simulink model "Forward_Kinematic"  (R2016a)
settings: Solver=VariableStepAuto  StartTime=0.0  StopTime=5  RelTol=1e-3
values from neighbouring files (symbols this model uses):
  l1 = 315    [FORWARD_KINEMATICS_DELTA_ROBOT.m]    (also in Inverse_Dynamic_Model.m = 0.1; Kinematic_Dimension.m = 0.315; inverse_kinematic.m = 0.1)
  phi = [phi1; phi2; phi3]    [Inverse_Dynamic_Model.m]    (also in Kinematic_Dimension.m; inverse_kinematic.m)
  r1 = 225    [FORWARD_KINEMATICS_DELTA_ROBOT.m]    (also in Inverse_Dynamic_Model.m = 0.35; Kinematic_Dimension.m = 0.225; inverse_kinematic.m = 0.35)
  r2 = 75    [FORWARD_KINEMATICS_DELTA_ROBOT.m]    (also in Inverse_Dynamic_Model.m = 0.35; Kinematic_Dimension.m = 0.075; inverse_kinematic.m = 0.35)
settings Model: Creator=computer  LastModifiedBy=computer
settings DataIOCC: SaveFormat=Array

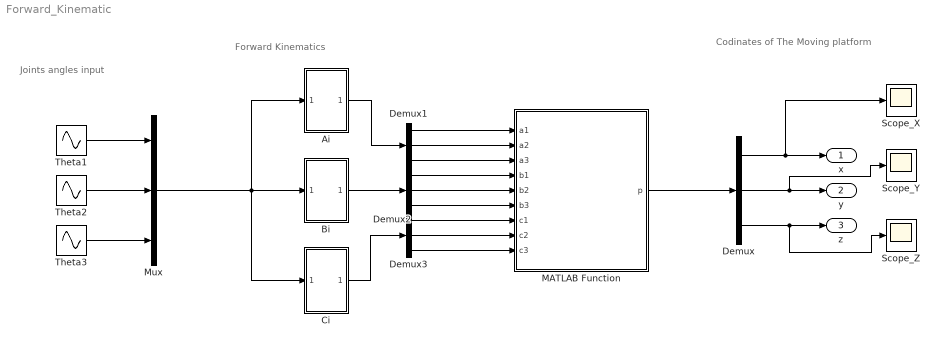
== system Forward_Kinematic ==
  note: Forward Kinematics
  note: Codinates of The Moving platform
  note: Joints angles input
  Ai : Subsystem
  Bi : Subsystem
  Ci : Subsystem
  Demux{,1..3} (4 alike) : Demux  Outputs=3
  MATLAB Function : MATLAB Function  TreatAsAtomicUnit=on
  Mux : Mux  Inputs=3
  Scope_X : Scope
  Scope_Y : Scope
  Scope_Z : Scope
  Theta1 : Sin  Frequency=1.5  SampleTime=0
  Theta2 : Sin  Amplitude=0.5  Bias=pi/8  Frequency=pi/2  SampleTime=0
  Theta3 : Sin  Amplitude=0.5  Frequency=pi  SampleTime=0
  x : Outport
  y : Outport  Port=2
  z : Outport  Port=3
  wires:
  Theta2/1 -> Mux/2
  Theta1/1 -> Mux/1
  Theta3/1 -> Mux/3
  Demux/3 -> Scope_Z/1, z/1
  Demux/2 -> y/1, Scope_Y/1
  Demux/1 -> Scope_X/1, x/1
  MATLAB Function/1(p) -> Demux/1
  Bi/1(Out1) -> Demux2/1
  Demux3/2 -> MATLAB Function/8(c2)
  Demux3/1 -> MATLAB Function/7(c1)
  Mux/1 -> Ci/1(In1), Ai/1(In1), Bi/1(In1)
  Demux3/3 -> MATLAB Function/9(c3)
  Demux2/1 -> MATLAB Function/4(b1)
  Demux2/3 -> MATLAB Function/6(b3)
  Ai/1(Out1) -> Demux1/1
  Demux2/2 -> MATLAB Function/5(b2)
  Ci/1(Out1) -> Demux3/1
  Demux1/2 -> MATLAB Function/2(a2)
  Demux1/1 -> MATLAB Function/1(a1)
  Demux1/3 -> MATLAB Function/3(a3)

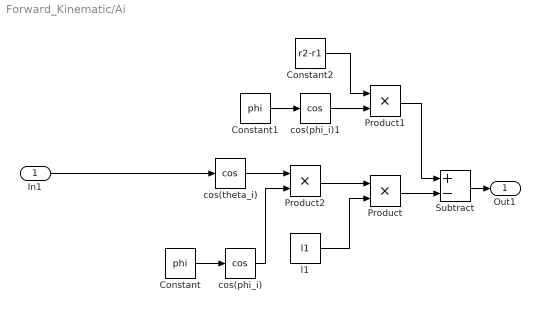
== system Forward_Kinematic/Ai ==
  In1 : Inport
  Constant : Constant  Value=phi
  Constant1 : Constant  Value=phi
  Constant2 : Constant  Value=r2-r1
  Product : Product
  Product1 : Product
  Product2 : Product
  Subtract : Sum  Inputs=+-
  cos(phi_i) : Trigonometry  Operator=cos
  cos(phi_i)1 : Trigonometry  Operator=cos
  cos(theta_i) : Trigonometry  Operator=cos
  l1 : Constant  Value=l1
  Out1 : Outport
  wires:
  Product1/1 -> Subtract/1
  Product/1 -> Subtract/2
  Constant1/1 -> cos(phi_i)1/1
  Subtract/1 -> Out1/1
  cos(phi_i)/1 -> Product2/2
  cos(phi_i)1/1 -> Product1/2
  Product2/1 -> Product/1
  cos(theta_i)/1 -> Product2/1
  Constant/1 -> cos(phi_i)/1
  l1/1 -> Product/2
  Constant2/1 -> Product1/1
  In1/1 -> cos(theta_i)/1

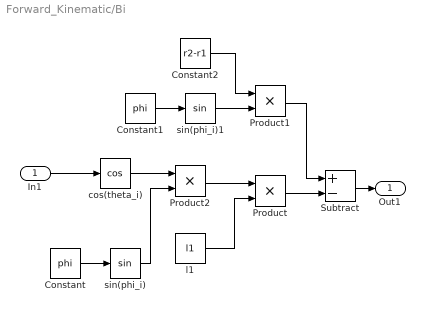
== system Forward_Kinematic/Bi ==
  In1 : Inport
  Constant : Constant  Value=phi
  Constant1 : Constant  Value=phi
  Constant2 : Constant  Value=r2-r1
  Product : Product
  Product1 : Product
  Product2 : Product
  Subtract : Sum  Inputs=+-
  cos(theta_i) : Trigonometry  Operator=cos
  l1 : Constant  Value=l1
  sin(phi_i) : Trigonometry
  sin(phi_i)1 : Trigonometry
  Out1 : Outport
  wires:
  In1/1 -> cos(theta_i)/1
  Constant2/1 -> Product1/1
  l1/1 -> Product/2
  Constant/1 -> sin(phi_i)/1
  cos(theta_i)/1 -> Product2/1
  Product2/1 -> Product/1
  sin(phi_i)1/1 -> Product1/2
  sin(phi_i)/1 -> Product2/2
  Subtract/1 -> Out1/1
  Constant1/1 -> sin(phi_i)1/1
  Product/1 -> Subtract/2
  Product1/1 -> Subtract/1

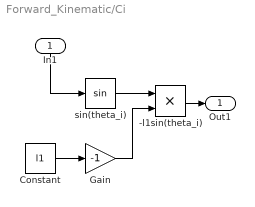
== system Forward_Kinematic/Ci ==
  In1 : Inport
  -l1sin(theta_i) : Product
  Constant : Constant  Value=l1
  Gain : Gain  Gain=-1
  sin(theta_i) : Trigonometry
  Out1 : Outport
  wires:
  Gain/1 -> -l1sin(theta_i)/2
  Constant/1 -> Gain/1
  In1/1 -> sin(theta_i)/1
  -l1sin(theta_i)/1 -> Out1/1
  sin(theta_i)/1 -> -l1sin(theta_i)/1

== matlab function Forward_Kinematic/MATLAB Function ==
  data: p output; a1 input; a2 input; a3 input; b1 input; b2 input; b3 input; c1 input; c2 input; c3 input
function p = equasol(a1, a2, a3, b1, b2, b3, c1, c2, c3)
%#codegen
 coder.extrinsic('solequa'); 
 p = zeros(3,1);
 p = solequa(a1, a2, a3, b1, b2, b3, c1, c2, c3);
